simulink model "program_control"  (R2022b)
settings: Solver=VariableStepAuto  StartTime=0.0  StopTime=1  RelTol=1e-3
settings Model: Creator=anver  LastModifiedBy=anver

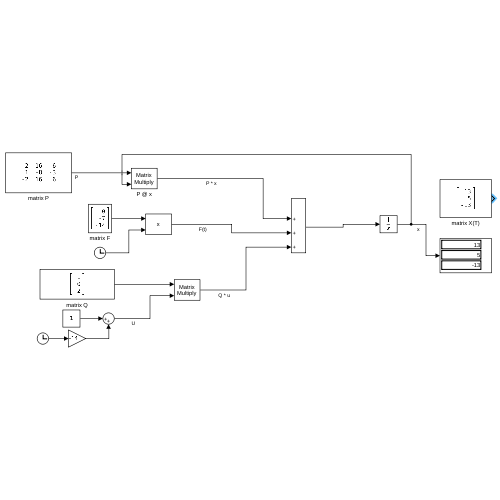
[thumbnail: Simulink's stored preview of the top-level diagram]
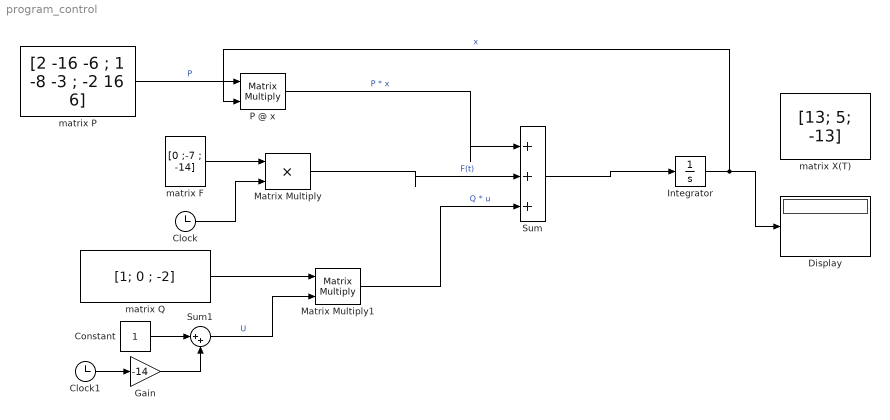
== system program_control ==
  Clock : Clock
  Clock1 : Clock
  Constant : Constant
  Display : Display
  Gain : Gain  Gain=-14
  Integrator : Integrator  InitialCondition=[2; 0; -1]
  Matrix Multiply : Product
  Matrix Multiply1 : Product  Multiplication=Matrix(*)
  P @ x : Product  Multiplication=Matrix(*)
  Sum : Sum  Inputs=|+++
  Sum1 : Sum  Inputs=|++
  matrix F : Constant  Value=[0 ;-7 ; -14]  VectorParams1D=off
  matrix P : Constant  Value=[2 -16 -6 ; 1 -8 -3 ; -2 16 6]  VectorParams1D=off
  matrix Q : Constant  Value=[1; 0 ; -2]  VectorParams1D=off
  matrix X(T) : Constant  Value=[13; 5; -13]  VectorParams1D=off
  wires:
  Integrator/1 -> P @ x/2, Display/1  "x"
  P @ x/1 -> Sum/1  "P * x"
  matrix F/1 -> Matrix Multiply/1
  Clock/1 -> Matrix Multiply/2
  matrix Q/1 -> Matrix Multiply1/1
  Constant/1 -> Sum1/1
  Gain/1 -> Sum1/2
  Clock1/1 -> Gain/1
  Sum1/1 -> Matrix Multiply1/2  "U"
  Sum/1 -> Integrator/1
  Matrix Multiply1/1 -> Sum/3  "Q * u"
  Matrix Multiply/1 -> Sum/2  "F(t)"
  matrix P/1 -> P @ x/1  "P"
